simulink model "Puncture_Through_Wall_r2007a"  (Simulink 6.0)
settings: Solver=ode1  StartTime=0.0  StopTime=inf  FixedStep=0.001  RelTol=1e-3
undefined symbols (not defined in the file): HIL, qc_get_step_size
libraries: simulink x5, quarc_library x4, vrlib x1
settings Model: Creator=RSamra  LastModifiedBy=ajavid  SimulationMode=external  ExtModeTrigDuration=10000
settings SolverCC: PositivePriorityOrder=on
settings OptimizationCC: InlineInvariantSignals=off  ExpressionDepthLimit=2147483647  SimCompilerOptimization=Off
settings DebuggingCC: SignalResolutionControl=UseLocalSettings  FcnCallInpInsideContextMsg=Use local settings  StateNameClashWarn=warning  StrictBusMsg=Warning
settings HardwareCC: TargetHWDeviceType=32-bit Generic
settings RTWCC: SystemTargetFile=quarc_windows.tlc  TemplateMakefile=quarc_default_tmf  Description=QuaRC Win32 Target  ProcessScript=quarc_windows_make_rtw_hook  RTWCompilerOptimization=Off
settings CodeAppCC: CustomSymbolStrType=$N$R$M
settings STFCustomTargetCC: TargetFcnLib=ansi_tfl_tmw.mat  TargetPreCompLibLocation=C:\DOCUME~1\ALLUSE~1\APPLIC~1\QuaRC\lib\2007b\windows\release  GenFloatMathFcnCalls=ANSI_C  SystemTargetFile=quarc_windows.tlc
settings GRTTargetCC: TargetPreCompLibLocation=C:\DOCUME~1\ALLUSE~1\APPLIC~1\QuaRC\lib\2007b\windows\release  CompOptLevelCompliant=off  MatFileLogging=off  ExtMode=on  ExtModeMexFile=quarc_comm

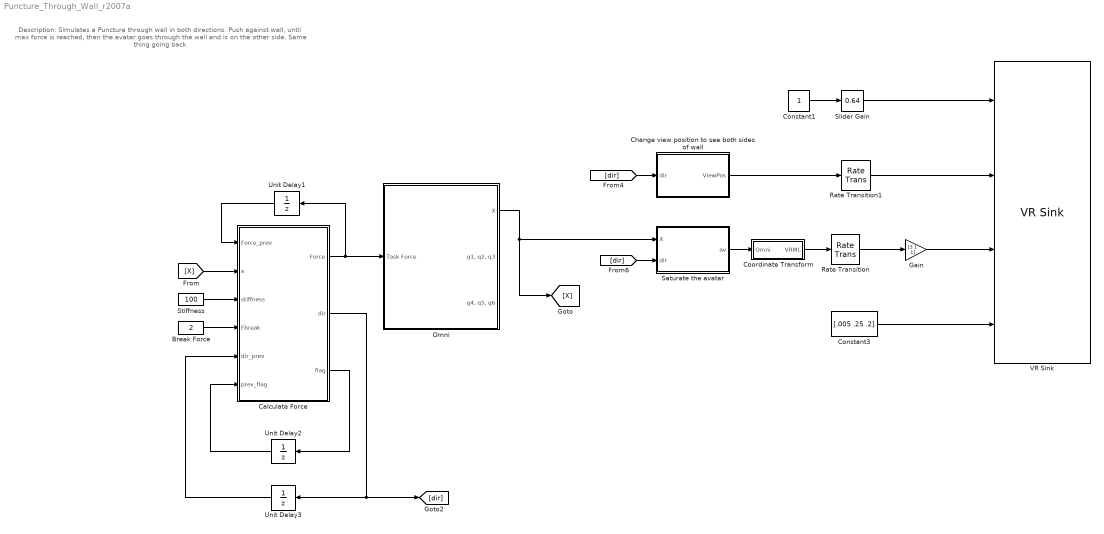
== system Puncture_Through_Wall_r2007a ==
  note: Description: Simulates a Puncture through wall in both directions.
      | Push against wall, until max force is reached, then the avatar goes through the wall and is on the other side. Same thing going back
  Break Force : Constant  Value=2  OutDataType=sfix(16)  OutScaling=2^0
  Calculate Force : Stateflow chart
      settings: PermitHierarchicalResolution=ParametersOnly
  Change view position to see both sides of wall : Subsystem
  Constant1 : Constant  OutDataType=sfix(16)  OutScaling=2^0
  Constant3 : Constant  Value=[.005 .25 .2]  OutDataType=sfix(16)  OutScaling=2^0
  Coordinate Transform : Subsystem
  Gain : Gain  Gain=[3 1 1]  ParameterDataType=sfix(16)  ParameterScaling=2^0  OutDataType=sfix(16)  OutScaling=2^0
  Omni : Subsystem
  Rate Transition : RateTransition
  Rate Transition1 : RateTransition
  Saturate the avatar : Subsystem
  Slider Gain : simulink/Math Operations/Slider Gain  SystemSampleTime=-1  low=0  gain=0.64  high=2
  Stiffness : Constant  Value=100  OutDataType=sfix(16)  OutScaling=2^0
  Unit Delay1 : UnitDelay  Orientation=left  X0=[0;0;0]  SampleTime=-1
  Unit Delay2 : UnitDelay  Orientation=left  SampleTime=-1
  Unit Delay3 : UnitDelay  Orientation=left  X0=1  SampleTime=-1
  VR Sink : vrlib/VR Sink  SampleTime=0.1  ViewEnable=on  RemoteChange=off  RemoteView=on  FieldsWritten=MyView.fieldOfView.1.1.double#MyView.position.3.1.double#Avatar.translation.3.1.double#Wall.scale.3.1.double  WorldFileName=PunctureThroughWall.WRL  WorldDescription=PunctureThroughWall  AutoView=on  VideoDimensions=[]  FigureProperties="{'Position', 'Name', 'Viewpoint', 'CameraBound', 'CameraDirection', 'CameraPosition', 'CameraUpVector', 'ZoomFactor', 'Antialiasing', 'Headlight', 'Lighting', 'NavPanel', 'StatusBar', 'ToolBar', 'Textures', 'Transparency', 'Wireframe', 'NavZones', 'NavMode', 'NavSpeed', 'Record2DCompressMethod', 'Record2DCompressQuality', 'Record2D', 'Record2DFileName', 'Record2DFPS'; [5.0000000000000000e+000  9.2000000000000000e+001  5.7600000000000000e+002  3.8000000000000000e+002], 'PunctureThroughWall', '_untitled_1', 'on', [0.0000000000000000e+000  0.0000000000000000e+000 -1.0000000000000000e+000], [0.0000000000000000e+000  0.0000000000000000e+000  0.0000000000000000e+000], [0.0000000000000000e+000  1.0000000000000000e+000  0.0000000000000000e+000], [1.0000000000000000e+000], 'off', 'on', 'on', 'halfbar', 'off', 'on', 'on', 'on', 'off', 'off', 'fly', 'normal', 'auto', [7.5000000000000000e+001], 'off', '%f_anim_%n.avi', [1.5000000000000000e+001]}"
  wires:
  [X] -> Calculate Force/2(x)
  Calculate Force/1(Force) -> Unit Delay1/1, Omni/1(Task Force)
  Stiffness/1 -> Calculate Force/3(stiffness)
  Constant1/1 -> Slider Gain/1
  [dir] -> Change view position to see both sides of wall/1(dir)
  [dir] -> Saturate the avatar/2(dir)
  Coordinate Transform/1("VRML ") -> Rate Transition/1
  Omni/1(X) -> Saturate the avatar/1(X), [X]
  Slider Gain/1 -> VR Sink/1
  Constant3/1 -> VR Sink/4
  Rate Transition1/1 -> VR Sink/2
  Unit Delay1/1 -> Calculate Force/1(Force_prev)
  Change view position to see both sides of wall/1(ViewPos) -> Rate Transition1/1
  Saturate the avatar/1(av) -> Coordinate Transform/1(Omni)
  Break Force/1 -> Calculate Force/4(Fbreak)
  Calculate Force/2(dir) -> Unit Delay3/1, [dir]
  Unit Delay3/1 -> Calculate Force/5(dir_prev)
  Calculate Force/3(flag) -> Unit Delay2/1
  Unit Delay2/1 -> Calculate Force/6(prev_flag)
  Rate Transition/1 -> Gain/1
  Gain/1 -> VR Sink/3

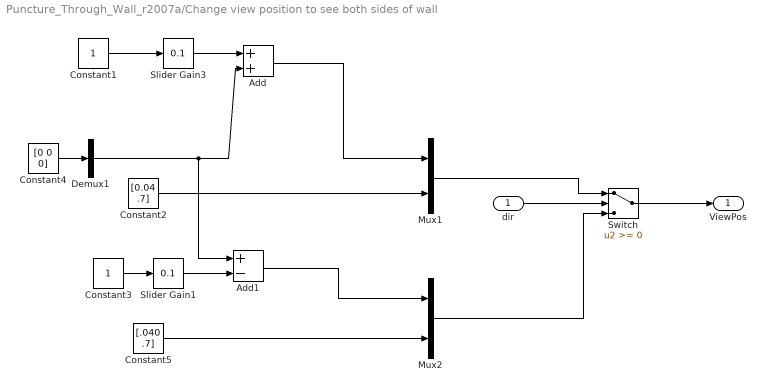
== system Puncture_Through_Wall_r2007a/Change view position to see both sides of wall ==
  dir : Inport
  Add : Sum  OutDataType=sfix(16)  OutScaling=2^-10
  Add1 : Sum  Inputs=+-  OutDataType=sfix(16)  OutScaling=2^-10
  Constant1 : Constant  OutDataType=sfix(16)  OutScaling=2^0
  Constant2 : Constant  Value=[0.04 .7]  OutDataType=sfix(16)  OutScaling=2^0
  Constant3 : Constant  OutDataType=sfix(16)  OutScaling=2^0
  Constant4 : Constant  Value=[0 0 0]  OutDataType=sfix(16)  OutScaling=2^0
  Constant5 : Constant  Value=[.040 .7]  OutDataType=sfix(16)  OutScaling=2^0
  Demux1 : Demux  Outputs=3
  Mux1 : Mux  Inputs=[1 2]
  Mux2 : Mux  Inputs=[1 2]
  Slider Gain1 : simulink/Math Operations/Slider Gain  SystemSampleTime=-1  low=0  gain=0.1  high=1
  Slider Gain3 : simulink/Math Operations/Slider Gain  SystemSampleTime=-1  low=0  gain=0.1  high=1
  Switch : Switch
  ViewPos : Outport
  wires:
  Constant2/1 -> Mux1/2
  Demux1/2 -> Add/2, Add1/1
  Mux1/1 -> Switch/1
  Constant5/1 -> Mux2/2
  Mux2/1 -> Switch/3
  dir/1 -> Switch/2
  Constant4/1 -> Demux1/1
  Switch/1 -> ViewPos/1
  Constant1/1 -> Slider Gain3/1
  Slider Gain3/1 -> Add/1
  Add/1 -> Mux1/1
  Constant3/1 -> Slider Gain1/1
  Slider Gain1/1 -> Add1/2
  Add1/1 -> Mux2/1

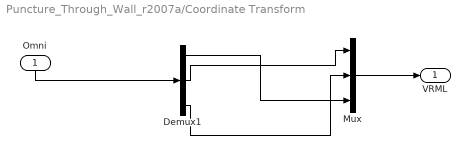
== system Puncture_Through_Wall_r2007a/Coordinate Transform ==
  Omni : Inport  Orientation=down
  Demux1 : Demux  Outputs=3
  Mux : Mux  Inputs=3
  "VRML " : Outport
  wires:
  Omni/1 -> Demux1/1
  Mux/1 -> "VRML "/1
  Demux1/1 -> Mux/3
  Demux1/2 -> Mux/1
  Demux1/3 -> Mux/2

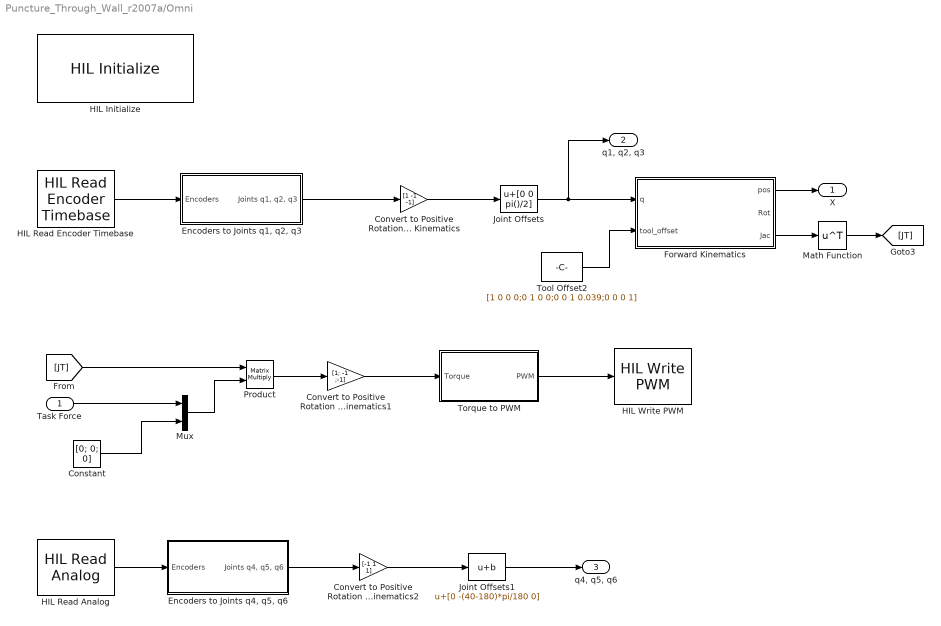
== system Puncture_Through_Wall_r2007a/Omni ==
  Task Force : Inport
  Constant : Constant  Value=[0; 0; 0]  VectorParams1D=off  OutDataType=sfix(16)  OutScaling=2^0
  Convert to Positive Rotation Convension Used in Kinematics : Gain  Gain=[1 -1 -1]  ParameterDataType=sfix(16)  ParameterScaling=2^0  OutDataType=sfix(16)  OutScaling=2^0
  Convert to Positive Rotation Convension Used in Kinematics1 : Gain  Gain=[1; -1 ;-1]  ParameterDataType=sfix(16)  ParameterScaling=2^0  OutDataType=sfix(16)  OutScaling=2^0
  Convert to Positive Rotation Convension Used in Kinematics2 : Gain  Gain=[-1 1 1]  ParameterDataType=sfix(16)  ParameterScaling=2^0  OutDataType=sfix(16)  OutScaling=2^0
  "Encoders to Joints q1, q2, q3" : Subsystem
  "Encoders to Joints q4, q5, q6" : Subsystem
  "Forward Kinematics " : Stateflow chart
      settings: PermitHierarchicalResolution=ParametersOnly
  HIL Initialize : quarc_library/Data Acquisition/Generic/Configuration/HIL Initialize  object_name=HIL-1  board_type=phantom_omni  board_number=0  active=on  hardware_clocks=[]  clock_modes=[]  set_clock_params_at_start=off  set_clock_params_at_switch_in=off  analog_input_channels=0:1  analog_input_maximums=10  analog_input_minimums=-10  set_analog_input_params_at_start=off  set_analog_input_params_at_switch_in=off  analog_output_channels=[]  analog_output_maximums=[]  analog_output_minimums=[]  initial_analog_outputs=[]  final_analog_outputs=[]  watchdog_analog_outputs=0  set_analog_output_params_at_start=off  set_analog_output_params_at_switch_in=off  set_analog_outputs_at_start=off  set_analog_outputs_at_switch_in=off  set_analog_outputs_at_terminate=off  set_analog_outputs_at_switch_out=off  set_analog_outputs_on_watchdog=off  digital_input_channels=[]  digital_output_channels=[]  initial_digital_outputs=[]  final_digital_outputs=[]  watchdog_digital_outputs=0  set_digital_outputs_at_start=off  set_digital_outputs_at_switch_in=off  set_digital_outputs_at_terminate=off  set_digital_outputs_at_switch_out=off  set_digital_outputs_on_watchdog=off  encoder_channels=0:2  quadrature=[]  encoder_filter_frequency=[]  initial_encoder_counts=0  set_encoder_params_at_start=off  set_encoder_params_at_switch_in=off  set_encoder_counts_at_start=off  set_encoder_counts_at_switch_in=off  pwm_channels=0:2  pwm_modes=[]  pwm_frequency=[]  initial_pwm_outputs=0  final_pwm_outputs=0  watchdog_pwm_outputs=0  set_pwm_params_at_start=off  set_pwm_params_at_switch_in=off  set_pwm_outputs_at_start=on  set_pwm_outputs_at_switch_in=off  set_pwm_outputs_at_terminate=on  set_pwm_outputs_at_switch_out=off  set_pwm_outputs_on_watchdog=off  other_output_channels=[]  initial_other_outputs=[]  final_other_outputs=[]  watchdog_other_outputs=0  set_other_outputs_at_start=off  set_other_outputs_at_switch_in=off  set_other_outputs_at_terminate=off  set_other_outputs_at_switch_out=off  set_other_outputs_on_watchdog=off
  HIL Read Analog : quarc_library/Data Acquisition/Generic/Immediate I//O/HIL Read Analog  object_name=HIL-1  channels=[0:2]  sample_time=qc_get_step_size  active=on  vector_output=on
  HIL Read Encoder Timebase : quarc_library/Data Acquisition/Generic/Timebases/HIL Read Encoder Timebase  object_name=HIL-1  clock=0  channels=0:2  samples_in_buffer=max(ceil(1/qc_get_step_size), 1)  active=on  vector_output=on  data_type_mode=Inherit via back propagation  data_type=double
  HIL Write PWM : quarc_library/Data Acquisition/Generic/Immediate I//O/HIL Write PWM  object_name=HIL-1  channels=0:2  sample_time=-1  active=off  vector_input=on
      settings: AttributesFormatString=(%<object_name>)
  Joint Offsets : Bias  Bias=[0 0 pi()/2]
  Joint Offsets1 : Bias  Bias=[0 -(40-180)*pi/180 0]  SaturateOnIntegerOverflow=on
  Math Function : Math  Operator=transpose  OutDataType=sfix(16)  OutScaling=2^0  SaturateOnIntegerOverflow=on
  Mux : Mux  Inputs=2
  Product : Product  Multiplication=Matrix(*)  OutDataType=sfix(16)  OutScaling=2^0  RndMeth=Zero
  Tool Offset2 : Constant  Value=[1 0 0 0;0 1 0 0;0 0 1 0.039;0 0 0 1]  VectorParams1D=off  OutDataType=sfix(16)  OutScaling=2^0
  Torque to PWM : Subsystem
  X : Outport
  "q1, q2, q3" : Outport  Port=2
  "q4, q5, q6" : Outport  Port=3
  wires:
  Tool Offset2/1 -> "Forward Kinematics "/2(tool_offset)
  Math Function/1 -> [JT]
  "Forward Kinematics "/3(Jac) -> Math Function/1
  [JT] -> Product/1
  Torque to PWM/1(PWM) -> HIL Write PWM/1
  "Forward Kinematics "/1(pos) -> X/1
  Constant/1 -> Mux/2
  Task Force/1 -> Mux/1
  Mux/1 -> Product/2
  "Encoders to Joints q1, q2, q3"/1("Joints q1, q2, q3") -> Convert to Positive Rotation Convension Used in Kinematics/1
  Convert to Positive Rotation Convension Used in Kinematics/1 -> Joint Offsets/1
  Convert to Positive Rotation Convension Used in Kinematics1/1 -> Torque to PWM/1(Torque)
  Product/1 -> Convert to Positive Rotation Convension Used in Kinematics1/1
  Joint Offsets/1 -> "Forward Kinematics "/1(q), "q1, q2, q3"/1
  HIL Read Encoder Timebase/1 -> "Encoders to Joints q1, q2, q3"/1(Encoders)
  HIL Read Analog/1 -> "Encoders to Joints q4, q5, q6"/1(Encoders)
  Convert to Positive Rotation Convension Used in Kinematics2/1 -> Joint Offsets1/1
  "Encoders to Joints q4, q5, q6"/1("Joints q4, q5, q6") -> Convert to Positive Rotation Convension Used in Kinematics2/1
  Joint Offsets1/1 -> "q4, q5, q6"/1

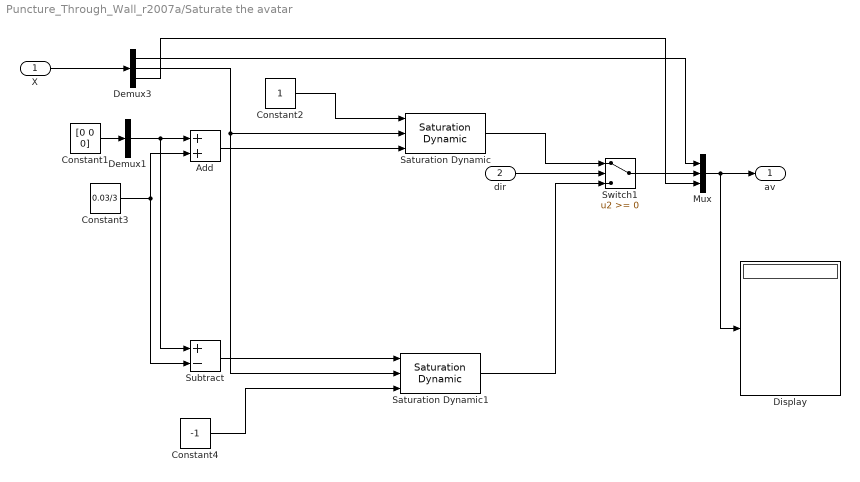
== system Puncture_Through_Wall_r2007a/Saturate the avatar ==
  X : Inport
  dir : Inport  Port=2
  Add : Sum  OutDataType=sfix(16)  OutScaling=2^-10
  Constant1 : Constant  Value=[0 0 0]  OutDataType=sfix(16)  OutScaling=2^0
  Constant2 : Constant  OutDataType=sfix(16)  OutScaling=2^0
  Constant3 : Constant  Value=0.03/3  OutDataType=sfix(16)  OutScaling=2^0
  Constant4 : Constant  Value=-1  OutDataType=sfix(16)  OutScaling=2^0
  Demux1 : Demux  Outputs=3
  Demux3 : Demux  Outputs=3
  Display : Display
  Mux : Mux  Inputs=3
  Saturation Dynamic : simulink/Discontinuities/Saturation Dynamic  SystemSampleTime=-1  OutDataType=sfix(16)  OutScaling=2^-10  DoSatur=off
  Saturation Dynamic1 : simulink/Discontinuities/Saturation Dynamic  SystemSampleTime=-1  OutDataType=sfix(16)  OutScaling=2^-10  DoSatur=off
  Subtract : Sum  Inputs=+-  OutDataType=sfix(16)  OutScaling=2^-10
  Switch1 : Switch
  av : Outport
  wires:
  Constant1/1 -> Demux1/1
  dir/1 -> Switch1/2
  Add/1 -> Saturation Dynamic/3
  X/1 -> Demux3/1
  Demux3/2 -> Saturation Dynamic/2, Saturation Dynamic1/2
  Constant2/1 -> Saturation Dynamic/1
  Saturation Dynamic/1 -> Switch1/1
  Constant3/1 -> Add/2, Subtract/2
  Demux1/2 -> Add/1, Subtract/1
  Subtract/1 -> Saturation Dynamic1/1
  Constant4/1 -> Saturation Dynamic1/3
  Saturation Dynamic1/1 -> Switch1/3
  Mux/1 -> av/1, Display/1
  Switch1/1 -> Mux/2
  Demux3/1 -> Mux/1
  Demux3/3 -> Mux/3

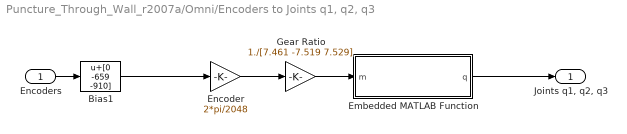
== system Puncture_Through_Wall_r2007a/Omni/Encoders to Joints q1, q2, q3 ==
  Encoders : Inport
  Bias1 : Bias  Bias=[0 -659 -910]
  Embedded MATLAB Function : Stateflow chart
      settings: PermitHierarchicalResolution=ParametersOnly
  Encoder : Gain  Gain=2*pi/2048  ParameterDataType=sfix(16)  ParameterScaling=2^0  OutDataType=sfix(16)  OutScaling=2^0
  Gear Ratio : Gain  Gain=1./[7.461 -7.519 7.529]  ParameterDataType=sfix(16)  ParameterScaling=2^0  OutDataType=sfix(16)  OutScaling=2^0
  "Joints q1, q2, q3" : Outport
  wires:
  Embedded MATLAB Function/1(q) -> "Joints q1, q2, q3"/1
  Encoders/1 -> Bias1/1
  Encoder/1 -> Gear Ratio/1
  Gear Ratio/1 -> Embedded MATLAB Function/1(m)
  Bias1/1 -> Encoder/1

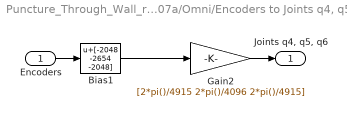
== system Puncture_Through_Wall_r2007a/Omni/Encoders to Joints q4, q5, q6 ==
  Encoders : Inport
  Bias1 : Bias  Bias=[-2048 -2654 -2048]
  Gain2 : Gain  Gain=[2*pi()/4915 2*pi()/4096 2*pi()/4915]  ParameterDataType=sfix(16)  ParameterScaling=2^0  OutDataType=sfix(16)  OutScaling=2^0
  "Joints q4, q5, q6" : Outport
  wires:
  Bias1/1 -> Gain2/1
  Encoders/1 -> Bias1/1
  Gain2/1 -> "Joints q4, q5, q6"/1

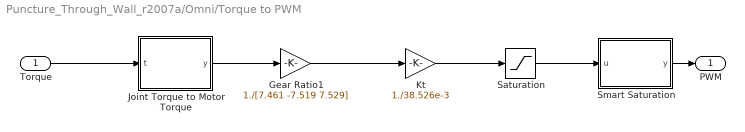
== system Puncture_Through_Wall_r2007a/Omni/Torque to PWM ==
  Torque : Inport
  Gear Ratio1 : Gain  Gain=1./[7.461 -7.519 7.529]  ParameterDataType=sfix(16)  ParameterScaling=2^0  OutDataType=sfix(16)  OutScaling=2^0
  Joint Torque to Motor Torque : Stateflow chart
      settings: PermitHierarchicalResolution=ParametersOnly
  Kt : Gain  Gain=1./38.526e-3  ParameterDataType=sfix(16)  ParameterScaling=2^0  OutDataType=sfix(16)  OutScaling=2^0
  Saturation : Saturate  UpperLimit=1.6  LowerLimit=-1.6
  Smart Saturation : Stateflow chart
      settings: PermitHierarchicalResolution=ParametersOnly
  PWM : Outport
  wires:
  Torque/1 -> Joint Torque to Motor Torque/1(t)
  Smart Saturation/1(y) -> PWM/1
  Saturation/1 -> Smart Saturation/1(u)
  Kt/1 -> Saturation/1
  Gear Ratio1/1 -> Kt/1
  Joint Torque to Motor Torque/1(y) -> Gear Ratio1/1

== matlab function Calculate Force ==
  data: Force_prev input inherited; Force output inherited; x input inherited; dir output inherited; stiffness input inherited; Fbreak input inherited; dir_prev input inherited; prev_flag input inherited; flag output inherited
function [Force,dir,flag]= fcn(Force_prev,x,stiffness,Fbreak,dir_prev,prev_flag)
%DESCRIPTION---------------------------------------------------------------
%Determine the force. The magnitude of the force is penetration into the wall
%The direction of force depends on the which of the wall the avatar is on. 
%The wall is implemented in the x-z

%INPUTS--------------------------------------------------------------------
%Force_prev - force in the previous sample time
%x - position of the avatar
%stiffness - stiffness of wall
%Fbreak - force required to break the wall
%dir_prev - the side of the wall where the avatar was in the previous sample time
%dir_flag - the value of flag in the previous sample time. flag is 1 when 
%the wall is broken, flag is 0 when the wall is solid.
%OUTPUTS-------------------------------------------------------------------
%Force - magnitude and direction of force to be applied
%dir - the side of the wall where the avatar is. If the avatar is strictly
%on the left dir = -1, if avatar is strictly on the right, dir = 1, else the
%avatar is touching or penetrating the wall and keep the previous direction
% flag - flag is 1 when the wall is broken , flag is 0 when wall is solid


%The y coordinate of the left side of the wall
x1wall = 0 - .01;
%The y coordinate of teh right side of the wall
x2wall = 0 + .01;

%The y coordinate of the avatar
av = x(2);

%declare variables
dir = dir_prev;
touching = 0;
Force = [0;0;0];
flag = prev_flag

%If inside the wall or pushing agains the wall, touching = 1, else 0. touching
%indicates when the wall is being touched.
if (av >= x1wall && av <= x2wall) || ( sign(Force_prev(2)) == dir)
    touching = 1;
else
    touching = 0;
end

%if the wall is broken, keep its state as broken, until the avatar is completly
%on one side of teh wall and not inside it.
if prev_flag == 1
    flag = 1;
    if (av <x1wall || av >x2wall)
        flag = 0;
    end
end

% If the wall is solid and the avatar is touchign the wall
%Calcualte the force based on the side of the wall the avatar is.
if dir == -1 && touching && av > x1wall && flag == 0
    Force = dir*stiffness*[0;abs(av-x1wall);0];
elseif dir == 1 && touching && av < x2wall && flag == 0
    Force = dir*stiffness*[0;abs(av-x2wall);0];
end

%If force is above break force, change the status of the wall to broken
if abs(Force(2)) >= Fbreak
    flag = 1;
end

% if avatar is on the left, dir = -1, elseif avatar is on theright dir = 1

if av < x1wall
    dir = -1;
elseif av > x2wall
    dir = 1;
end

== matlab function Omni/Torque to PWM/Smart Saturation ==
  data: u input inherited; y output inherited size=3
function y = fcn(u)
% Smart Saturation: allows channels to go up to 1.6A 
% unless the total exceeds 2.2A in which case all channels
% are scaled so that the cumulative current is equal to 2.2A.

y = zeros(3,1);
MAX_CURRENT = 2.2; % Define the maximum cumulative current here

total = sum(abs(u));
if (total > MAX_CURRENT)
    y = MAX_CURRENT/total*u;
else
    y = u;
end

== matlab function Omni/Torque to PWM/Joint Torque to Motor Torque ==
  data: t input inherited; y output inherited
function y = fcn( t)
% Smart Saturation: allows channels to go up to 1.6A 
% unless the total exceeds 2.2A in which case all channels
% are scaled so that the cumulative current is equal to 2.2A.
y=[0 0 0]'

y(1)=t(1);
y(3)=t(3);
y(2)=t(2)-t(3);


end

== matlab function Omni/Forward Kinematics  ==
  data: pos output inherited; q input inherited; Rot output inherited; tool_offset input inherited; Jac output inherited
function [pos,Rot,Jac]    = fcn(q,tool_offset)
% This block supports the Embedded MATLAB subset.
% See the help menu for details. 

% Link lengths
L1 = .132;
L2 = .132;

%Define A-matrices
%A1= DH(a_i ,alpha_i    ,d_i    ,theta_i)
A1 = DH(0   ,-pi()/2    ,0      ,q(1));
A2 = DH(L1  ,0          ,0      ,q(2));
A3 = DH(L2   ,0     ,0     ,q(3)-pi/2);

%Define T Matrices
T01=A1;
T02=T01*A2;
T03=T02*A3;

%Axes of rotation in base coordinates. 

z0=[0 0 1]';
z1=T01(1:3,3);
z2=T02(1:3,3);

%Coordinate Frame origins in Base frame coordinates

p0=[0 0 0]';
p1=T01(1:3,4);
p2=T02(1:3,4);
p3=T03(1:3,4);


%tool_offset given with respect to frame 3.
T_tool=T03*tool_offset;
Rot=T03(1:3,1:3);
pos=T_tool(1:3,4);

%Formulation of the Jacobian

%%%%%%%%%%%%%%%%%%%%%%%%%%%%JACOBIAN%%%%%%%%%%%%%%%%%%%%%%%%
Jac = [cross(z0,(pos-p0)) cross(z1,(pos-p1)) cross(z2,(pos-p2))
    z0 z1 z2];

end

function A = DH(a_x, alpha_x, d_z, theta_z)

A_R_z = [cos(theta_z) -sin(theta_z) 0 0;
         sin(theta_z) cos(theta_z) 0 0;
         0 0 1 0;
         0 0 0 1];

A_T_z = [1 0 0 0;
         0 1 0 0;
         0 0 1 d_z;
         0 0 0 1];
     
  

A_T_x = [1 0 0 a_x;
         0 1 0 0;
         0 0 1 0;
         0 0 0 1];

A_R_x = [1 0 0 0;
         0 cos(alpha_x) -sin(alpha_x)  0;
         0 sin(alpha_x) cos(alpha_x) 0;
         0 0 0 1];

A = A_R_z*A_T_z*A_T_x*A_R_x;

end

== matlab function Omni/Encoders to Joints q1, q2, q3/Embedded MATLAB Function ==
  data: m input inherited; q output inherited
function q = Motors_2_Joints(m)
q = m;
q(1) = m(1);
q(2) = m(2);
q(3) = m(3) - m(2) -pi/2;
end
